simulink model "Mpu_SimpleGyroModel"  (R2015b)
settings: Solver=ode5  StartTime=0.0  StopTime=180  FixedStep=1/mpu_sampling_frequency  RelTol=1e-3
values from neighbouring files (symbols this model uses):
  mpu_gyro_noise_density = 0.01    [imu_settings.m]    (also in mpu_plot.m)
  mpu_gyro_sensitivity = 0.0610    (= 0.061)    [imu_settings.m]    (also in mpu_plot.m)
  mpu_sampling_frequency = 819.2    [adis_imu_settings.m]    (also in imu_settings.m = 200; mpu_plot.m = 200)
  mpu_w = 250    [imu_settings.m]    (also in mpu_plot.m)
  wn = gyroscope_wn    (= 17500)    [PrepCode.m]
  zeta = 0.5    [PrepCode.m]
libraries: simulink x1
settings Model: Creator=TOOsab  LastModifiedBy=TOOsab

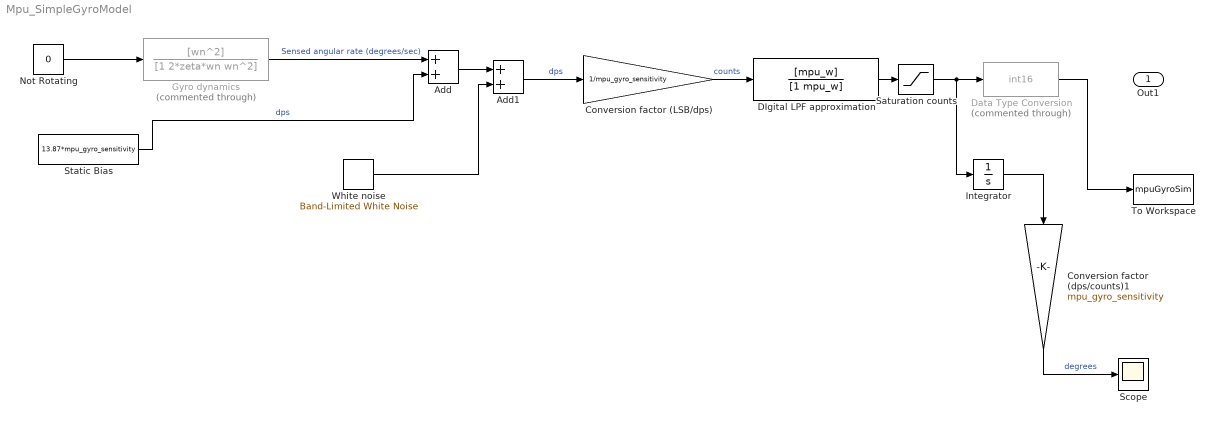
== system Mpu_SimpleGyroModel ==
  Add : Sum
  Add1 : Sum
  Conversion factor (LSB/dps) : Gain  Gain=1/mpu_gyro_sensitivity
  Conversion factor (dps/counts)1 : Gain  Gain=mpu_gyro_sensitivity
  DIgital LPF approximation : TransferFcn  Numerator=[mpu_w]  Denominator=[1 mpu_w]
  Data Type Conversion : DataTypeConversion  Commented=through  OutDataTypeStr=int16
  Gyro dynamics : TransferFcn  Commented=through  Numerator=[wn^2]  Denominator=[1 2*zeta*wn wn^2]
  Integrator : Integrator
  "Not Rotating " : Constant  Value=0
  "Saturation counts " : Saturate  UpperLimit=2^15  LowerLimit=-2^15
  Scope : Scope
  Static Bias : Constant  Value=13.87*mpu_gyro_sensitivity
  To Workspace : ToWorkspace  VariableName=mpuGyroSim  SampleTime=-1
  White noise : simulink/Sources/Band-Limited White Noise  Cov=[(mpu_gyro_noise_density)^2]  Ts=1/mpu_sampling_frequency  seed=[23341]
  Out1 : Outport
  wires:
  Conversion factor (LSB/dps)/1 -> DIgital LPF approximation/1  "counts"
  Static Bias/1 -> Add/2  "dps"
  Gyro dynamics/1 -> Add/1  "Sensed angular rate (degrees/sec)"
  White noise/1 -> Add1/2
  Add/1 -> Add1/1
  Add1/1 -> Conversion factor (LSB/dps)/1  "dps"
  DIgital LPF approximation/1 -> "Saturation counts "/1
  "Saturation counts "/1 -> Integrator/1, Data Type Conversion/1
  Data Type Conversion/1 -> To Workspace/1
  "Not Rotating "/1 -> Gyro dynamics/1
  Integrator/1 -> Conversion factor (dps/counts)1/1
  Conversion factor (dps/counts)1/1 -> Scope/1  "degrees"
